simulink model "Torsional_System"  (R2021b)
settings: Solver=daessc  StartTime=0.0  StopTime=10.0  FixedStep=.001  RelTol=1e-3  AbsTol=1e-3  EnableMultiTasking=on
undefined symbols (not defined in the file or in its folder): X, Y, Z
libraries: sm_lib x119, nesl_utility x21, slpidlib x1
(part 1 of 6)
settings Model: Creator=HP Owner  LastModifiedBy=acontr14
settings SolverCC: AutoScaleAbsTol=off  AlgebraicLoopSolver=TrustRegion
settings DataIOCC: LimitDataPoints=on  MaxDataPoints=10000
settings OptimizationCC: LifeSpan=inf
settings DebuggingCC: AllowSymbolicDim=off  SFUnexpectedBacktrackingDiag=warning  SFNoUnconditionalDefaultTransitionDiag=warning  SFExecutionAtInitializationDiag=none  SFMachineParentedDataDiag=warning  ArithmeticOperatorsInVariantConditions=warning
settings SFSimCC: SimUseLocalCustomCode=off  CustomCodeUndefinedFunction=UseInterfaceOnly
settings RTWCC: RTWUseLocalCustomCode=off
settings CodeAppCC: StateflowObjectComments=on
settings GRTTargetCC: TargetLangStandard=C89/C90 (ANSI)
settings ConfigComp: CovMetricSettings=dw  CovSaveCumulativeToWorkspaceVar=on  CovSaveSingleToWorkspaceVar=on  CovExternalEMLEnable=off  CovSFcnEnable=off
settings SimscapeCC: SimscapeLogType=all  SimscapeLogSimulationStatistics=on  SimscapeLogDataHistory=10000
settings ExplorerConfigSet: InternalSimMechanicsExplorerSettings="<ExplorerConfiguration><canonicalview>default</canonicalview><AnimationSetting><BasePlaybackSpeed>1.0</BasePlaybackSpeed><PlaybackSpeedFactor>1.0</PlaybackSpeedFactor></AnimationSetting><TilePanel><TileInfo><Tiles Columns=\"1\" Count=\"1\" Rows=\"1\"><Column Weight=\"1\"/><Row Weight=\"1\"/><Tile Height=\"1\" Width=\"1\" X=\"0\" Y=\"0\"/></Tiles></TileInfo><SceneInfo><SceneViewer><BGColor><R>1</R><G>1</G><B>1</B></BGColor><Camera><DoPerspective>off</DoPerspective><Position><X>-0.306662978347955806</X><Y>-0.940894619780998753</Y><Z>0.41893568511161039</Z></Position><Center><X>-0.0242515964490015445</X><Y>-0.0315683410689719945</Y><Z>0.11337140346540675</Z></Center><Up><X>0.08382140599557307</X><Y>0.29392098737897232</Y><Z>0.9521472706861559</Z></Up><ViewLimDist>1</ViewLimDist><YLim>0.135911061057100324</YLim><XLim>0.110417778795510582</XLim></Camera></SceneViewer></SceneInfo></TilePanel><MechEditorPanel><Cameras/><GfxPanelCameraMap/><VideoCreator><PlaybackSpeedRatio>1.0</PlaybackSpeedRatio><FrameRate>30</FrameRate><VideoFormat>Motion JPEG AVI</VideoFormat><FrameSize>auto</FrameSize></VideoCreator></MechEditorPanel></ExplorerConfiguration>"

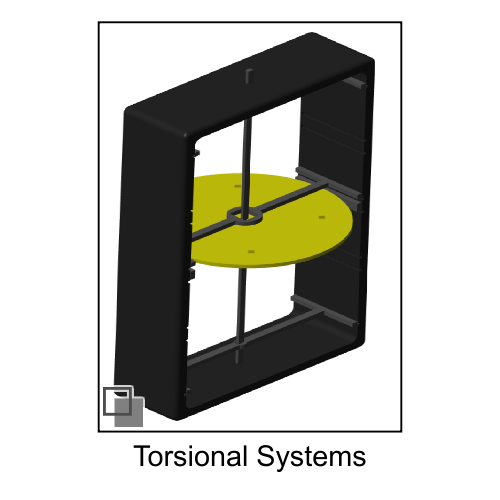
[thumbnail: Simulink's stored preview of the top-level diagram]
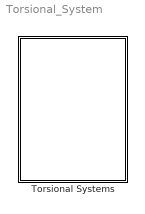
== system Torsional_System ==
  Torsional Systems : Subsystem  Variant=on  VariantControlMode=label  LabelModeActiveChoice=dof1PID

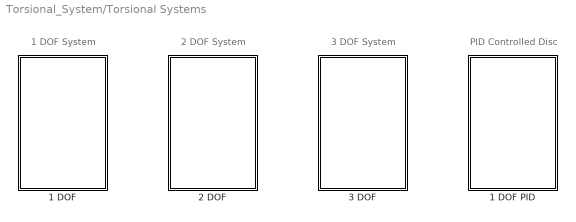
== system Torsional_System/Torsional Systems ==
  note: PID Controlled Disc
  note: 1 DOF System
  note: 2 DOF System
  note: 3 DOF System
  1 DOF : Subsystem  VariantControl=dof1  mask{materials=PLA, GG=3.5, b_den1=1.25, d_den=1.25, d=.000002, ll=106.800, load=off, lmass=5, dmass=15, pos1=50, zerodis=off, zero_forces=on, force_type=Harmonic, Force=2, Har_Force=2, freq=1}
      mask prompts: materials "Choose Material of Rod:"; GG "Shear Modulus (GPa):"; b_den1 "Density of Rod (g/cm^3):"; d_den "Density of Disc (g/cm^3):"; d "Rod Damping"; ll "Position of Disc (mm):"; load "Add load"; lmass "Load Mass (kg)"; dmass "Distance from Center (mm)"; pos1 "Initial Rotation of Disc (deg):"; zerodis "Zero Initial Displacement"; zero_forces "Zero Forces"; force_type "Force Response Type"; Force "Magnitude (N):"; Har_Force "Magnitude (N):"; freq "Frequency (rad/s):"
      mask init:
      | switch materials
      |     case 1
      |         G= 1; %GPa
      |         b_den= 1; %g/cm^3
      |     case 2
      |         G= 3.5;
      |         b_den= 1.24;
      |     case 3
      |         G= GG;
      |         b_den= b_den1;
      | end
      | switch force_type
      |     case 1
      |         Har_Force = 0;
      |         freq = 0;
      |     case 2
      |         Force = 0;
      | end
      | if zero_forces == 1
      |     Har_Force = 0;
      |     Force = 0;
      |     freq = 0;
      | end
      | if zerodis == 1
      |     pos1 = 0;
      | end
      | % l1=65e-3; l2=l1; l3=l1; l4=l1;
      | l=ll*10^-3;
      | l2=.2025-l;
      | G=G*10^9;
      | dd=2.25e-3;
      | k1=pi*G*dd^4/(32*l);
      | k2=(pi*G*dd^4/(32*l2));
      | % k3=(pi*G*dd^4/(32*l3));
      | kt1=k1+k2;
      | % kt2=k2+k3;
      | % kt3=2*k3;
      mask TypeOptions materials: Steel | PLA | Enter Material Properties
      mask Callback materials:
      | % Get the mask parameter values. This is a cell
      | %   array of character vectors.
      | maskStr = get_param(gcb,'materials');
      | 
      | % The pop-up menu is the first mask parameter.
      | %   Check the value selected in the pop-up
      | if strcmp(maskStr(1),'E'),
      | 
      |     % Set the visibility of both parameters on when
      |     %   User-defined is selected in the pop-up.
      | 
      |     set_param(gcb,'MaskVisibilities',{'on';'on';'on';'on';'on';'on';'on';'on';'on';'on';'on';'on';'on';'on';'on';'on'}),
      | 
      | else
      | 
      |     % Turn off the visibility of the Value field
      |     %   when User-defined is not selected.
      | 
      |     set_param(gcb,'MaskVisibilities',{'on';'off';'off';'on';'on';'on';'on';'on';'on';'on';'on';'on';'on';'on';'on';'on'}),
      | 
      |     % Set the character vector in the Values field equal to the
      |     % character vector selected in the Gain pop-up menu.
      | end
      mask Callback load:
      | load = get_param(gcb,'load');
      | if strcmp(load,'on')
      |     set_param('Torsional_System/Torsional Systems/1 DOF/Cylindrical Solid','Commented','off');
      |     set_param('Torsional_System/Torsional Systems/1 DOF/Rigid Transform2','Commented','off');
      | else
      |     set_param('Torsional_System/Torsional Systems/1 DOF/Cylindrical Solid','Commented','on');
      |     set_param('Torsional_System/Torsional Systems/1 DOF/Rigid Transform2','Commented','on');
      | end
      mask Callback zero_forces:
      | % Enable and disable parameters
      | 
      | % Get the value of the Enable Bias checkbox
      | % unchecked = 'off'
      | % checked = 'on'
      | enab = get_param(gcb,'zero_forces');
      | 
      | % Set the 'MaskEnables' property for each parameters
      | if strcmp(enab,'on')
      |     set_param(gcb,'MaskEnables',{'on','on','on','on','on','on','on','on','on','on','on','on','off','off','off','off'});
      | else
      |     set_param(gcb,'MaskEnables',{'on','on','on','on','on','on','on','on','on','on','on','on','on','on','on','on'});
      | end
      | 
      | % Note that the value of the bias is not handled here.
      | % See the Initialization tab
      mask TypeOptions force_type: Step | Harmonic
      mask DialogControl Control4 Prompt: Update Model
      mask DialogControl Control4 Callback: set_param(bdroot,'SimulationCommand','update')
      mask DialogControl Control3 Prompt: Run Simulation
      mask DialogControl Control3 Callback: set_param(bdroot,'SimulationCommand','start')
      mask DialogControl Control5 Prompt: Stop Simulation
      mask DialogControl Control5 Callback: set_param(bdroot,'SimulationCommand','stop')
      mask DialogControl Control2 Prompt: Open Position Plot
      mask DialogControl Control2 Callback: open(Simulink.BlockPath({'Torsional_System/Torsional Systems/1 DOF/Scope1'}))
      mask DialogControl Control7 Prompt: Open Frequency Plot
      mask DialogControl Control7 Callback:
      | disc1=evalin('base','out.disc1_pos');
      | time=evalin('base','out.tout');
      | 
      | Ts = time(2)-time(1);
      | fs = 1/Ts;
      | N = length(disc1);
      | 
      | Y1 = abs(fft(disc1)/N); % fft of cart1 data
      | Y1d = Y1(1:N/2+1); %single side spectrum
      | Y1d(2:end-1) = 2*Y1d(2:end-1); %amplitude adjustment
      | 
      | f = fs*(0:(N/2))/N; %create frequency vector
      | 
      | figure;
      | plot(f,Y1d); xlim([0 10]);
      mask DialogControl Container8 Prompt: Parameters
      mask DialogControl Container14 Prompt: Loading
      mask DialogControl Container13 Prompt: Free Response
      mask DialogControl Container17 Prompt: Force Response
      mask DialogControl Container18 Prompt: Step Response
      mask DialogControl Container19 Prompt: Harmonic Response
      mask Display: image('$imagefile'); % Use "Edit Image" on toolstrip to change.
  1 DOF PID : Subsystem  VariantControl=dof1PID  mask{materials=PLA, GG=3.5, b_den1=1.25, d_den=1.25, d=.000002, ll=106.800, load=off, lmass=5, dmass=37.0, pos1=50, zerodis=on, zero_forces=off, force_type=Pulse, Force=5, Har_Force=2, freq=1, Pulse_Force=2, Pulse_Period=3, Pulse_Width=5, PID_source=Square, sin_amp=30, sin_freq=1, squ_amp=50, squ_freq=.2, step_mag=30}
      mask prompts: materials "Choose Material of Rod:"; GG "Shear Modulus (GPa):"; b_den1 "Density of Rod (g/cm^3):"; d_den "Density of Disc (g/cm^3):"; d "Rod Damping"; ll "Position of Disc (mm):"; load "Add Load"; lmass "Load Mass (kg)"; dmass "Distance from Center (mm)"; pos1 "Initial Rotation of Disc (deg):"; zerodis "Zero Initial Displacement"; zero_forces "Zero Forces"; force_type "Force Response Type"; Force "Magnitude (N):"; Har_Force "Magnitude (N):"; freq "Frequency (rad/s):"; Pulse_Force "Magnitude (N):"; Pulse_Period "Period (sec):"; Pulse_Width "Pulse Width (% of period):"; PID_source "Angle Signal"; sin_amp "Amplitude (deg):"; sin_freq "Frequency (rad/sec):"; squ_amp "Amplitude (deg):"; squ_freq "Frequency (Hz):"; step_mag "Magnitude (deg):"
      mask init:
      | switch materials
      |     case 1
      |         G= 1; %GPa
      |         b_den= 1; %g/cm^3
      |     case 2
      |         G= 3.5;
      |         b_den= 1.24;
      |     case 3
      |         G= GG;
      |         b_den= b_den1;
      | end
      | switch force_type
      |     case 1
      |         Har_Force = 0;
      |         freq = 0;
      |         Pulse_Force = 0;
      |     case 2
      |         Force = 0;
      |         Pulse_Force = 0;
      |     case 3
      |         Har_Force = 0;
      |         freq = 0;
      |         Force = 0;
      | end
      | if zero_forces == 1
      |     Har_Force = 0;
      |     Force = 0;
      |     freq = 0;
      | end
      | if zerodis == 1
      |     pos1 = 0;
      | end
      | switch PID_source
      |     case 1
      |         set_param('Torsional_System/Torsional Systems/1 DOF PID/Sine Wave2','Commented','off');
      |         set_param('Torsional_System/Torsional Systems/1 DOF PID/Signal Generator','Commented','on');
      |         set_param('Torsional_System/Torsional Systems/1 DOF PID/Step2','Commented','on');
      |     case 2
      |         set_param('Torsional_System/Torsional Systems/1 DOF PID/Sine Wave2','Commented','on');
      |         set_param('Torsional_System/Torsional Systems/1 DOF PID/Signal Generator','Commented','off');
      |         set_param('Torsional_System/Torsional Systems/1 DOF PID/Step2','Commented','on');
      |     case 3
      |         set_param('Torsional_System/Torsional Systems/1 DOF PID/Sine Wave2','Commented','on');
      |         set_param('Torsional_System/Torsional Systems/1 DOF PID/Signal Generator','Commented','on');
      |         set_param('Torsional_System/Torsional Systems/1 DOF PID/Step2','Commented','off');
      | end
      | % l1=65e-3; l2=l1; l3=l1; l4=l1;
      | l=ll*10^-3;
      | l2=.2025-l;
      | G=G*10^9;
      | dd=2.25e-3;
      | k1=pi*G*dd^4/(32*l);
      | k2=(pi*G*dd^4/(32*l2));
      | % k3=(pi*G*dd^4/(32*l3));
      | kt1=k1+k2;
      | % kt2=k2+k3;
      | % kt3=2*k3;
      mask TypeOptions materials: Steel | PLA | Enter Material Properties
      mask Callback materials:
      | % Get the mask parameter values. This is a cell
      | %   array of character vectors.
      | maskStr = get_param(gcb,'materials');
      | 
      | % The pop-up menu is the first mask parameter.
      | %   Check the value selected in the pop-up
      | if strcmp(maskStr(1),'E'),
      | 
      |     % Set the visibility of both parameters on when
      |     %   User-defined is selected in the pop-up.
      | 
      |     set_param(gcb,'MaskVisibilities',{'on';'on';'on';'on';'on';'on';'on';'on';'on';'on';'on';'on';'on';'on';'on';'on';'on';'on';'on';'on';'on';'on';'on';'on';'on'}),
      | 
      | else
      | 
      |     % Turn off the visibility of the Value field
      |     %   when User-defined is not selected.
      | 
      |     set_param(gcb,'MaskVisibilities',{'on';'off';'off';'on';'on';'on';'on';'on';'on';'on';'on';'on';'on';'on';'on';'on';'on';'on';'on';'on';'on';'on';'on';'on';'on'}),
      | 
      |     % Set the character vector in the Values field equal to the
      |     % character vector selected in the Gain pop-up menu.
      | end
      mask Callback load:
      | load = get_param(gcb,'load');
      | if strcmp(load,'on')
      |     set_param('Torsional_System/Torsional Systems/1 DOF PID/Cylindrical Solid','Commented','off');
      |     set_param('Torsional_System/Torsional Systems/1 DOF PID/Rigid Transform9','Commented','off');
      |     set_param('Torsional_System/Torsional Systems/1 DOF PID/Cylindrical Solid1','Commented','off');
      |     set_param('Torsional_System/Torsional Systems/1 DOF PID/Rigid Transform7','Commented','off');
      | else
      |     set_param('Torsional_System/Torsional Systems/1 DOF PID/Cylindrical Solid','Commented','on');
      |     set_param('Torsional_System/Torsional Systems/1 DOF PID/Rigid Transform9','Commented','on');
      |     set_param('Torsional_System/Torsional Systems/1 DOF PID/Cylindrical Solid1','Commented','on');
      |     set_param('Torsional_System/Torsional Systems/1 DOF PID/Rigid Transform7','Commented','on');
      | end
      mask Callback zero_forces:
      | % Enable and disable parameters
      | 
      | % Get the value of the Enable Bias checkbox
      | % unchecked = 'off'
      | % checked = 'on'
      | enab = get_param(gcb,'zero_forces');
      | 
      | % Set the 'MaskEnables' property for each parameters
      | if strcmp(enab,'on')
      |     set_param(gcb,'MaskEnables',{'on','on','on','on','on','on','on','on','on','on','on','on','off','off','off','off','off','off','off','on','on','on','on','on','on'});
      | else
      |     set_param(gcb,'MaskEnables',{'on','on','on','on','on','on','on','on','on','on','on','on','on','on','on','on','on','on','on','on','on','on','on','on','on'});
      | end
      | 
      | % Note that the value of the bias is not handled here.
      | % See the Initialization tab
      mask TypeOptions force_type: Step | Harmonic | Pulse
      mask TypeOptions PID_source: Harmonic | Square | Constant
      mask DialogControl Control4 Prompt: Update Model
      mask DialogControl Control4 Callback: set_param(bdroot,'SimulationCommand','update')
      mask DialogControl Control3 Prompt: Run Simulation
      mask DialogControl Control3 Callback: set_param(bdroot,'SimulationCommand','start')
      mask DialogControl Control5 Prompt: Stop Simulation
      mask DialogControl Control5 Callback: set_param(bdroot,'SimulationCommand','stop')
      mask DialogControl Control2 Prompt: Open Position Plot
      mask DialogControl Control2 Callback: open(Simulink.BlockPath({'Torsional_System/Torsional Systems/1 DOF PID/Scope1'}))
      mask DialogControl Control7 Prompt: Open PID Controller
      mask DialogControl Control7 Callback: open(Simulink.BlockPath({'Torsional_System/Torsional Systems/1 DOF PID/PID Controller'}))
      mask DialogControl Container8 Prompt: Parameters
      mask DialogControl Container14 Prompt: Loading
      mask DialogControl Container13 Prompt: Free Response
      mask DialogControl Container17 Prompt: Force Response
      mask DialogControl Container18 Prompt: Step Response
      mask DialogControl Container19 Prompt: Harmonic Response
      mask DialogControl Container23 Prompt: Pulse
      mask DialogControl Container16 Prompt: PID Desired Angle
      mask DialogControl Container20 Prompt: Harmonic
      mask DialogControl Container21 Prompt: Square
      mask DialogControl Container22 Prompt: Constant
      mask Display: image('$imagefile'); % Use "Edit Image" on toolstrip to change.
  2 DOF : Subsystem  VariantControl=dof2  mask{materials=PLA, GG=3.5, b_den1=1.25, d_den=1.25, d=.000002, ll1=45.600, ll2=163.0, load=off, lmass=5, dmass=15, pos1=15, pos2=30, zerodis=off, zero_forces=on, force_type=Step, Force_m1=0, Force_m2=0, Har_Force_m1=0, freq_m1=0, Har_Force_m2=0, freq_m2=0}
      mask prompts: materials "Choose Material of Rod:"; GG "Shear Modulus (GPa):"; b_den1 "Density of Rod (g/cm^3):"; d_den "Density of Discs (g/cm^3):"; d "Rod Damping"; ll1 "Position of Disc 1 (mm):"; ll2 "Position of Disc 2 (mm):"; load "Add load"; lmass "Load Mass (kg)"; dmass "Distance from Center (mm)"; pos1 "Initial Rotation of Disc 1 (deg):"; pos2 "Initial Rotation of Disc 2 (deg):"; zerodis "Zero Initial Displacement"; zero_forces "Zero Forces"; force_type "Force Response Type"; Force_m1 "Magnitude  on Disc 1 (N):"; Force_m2 "Magnitude  on Disc 2 (N):"; Har_Force_m1 "Magnitude on Disc 1 (N):"; freq_m1 "Frequency on Disc 1 (rad/s):"; Har_Force_m2 "Magnitude on Disc 2 (N):"; freq_m2 "Frequency on Disc 2 (rad/s):"
      mask init:
      | switch materials
      |     case 1
      |         G= 1; %GPa
      |         b_den= 1; %g/cm^3
      |     case 2
      |         G= 3.5;
      |         b_den= 1.24;
      |     case 3
      |         G= GG;
      |         b_den= b_den1;
      | end
      | switch force_type
      |     case 1
      |         Har_Force_m1 = 0;
      |         freq_m1 = 0;
      |         Har_Force_m2 = 0;
      |         freq_m2 = 0;
      |     case 2
      |         Force_m1 = 0;
      |         Force_m2 = 0;
      | end
      | if zero_forces == 1
      |     Har_Force_m1 = 0;
      |     freq_m1 = 0;
      |     Har_Force_m2 = 0;
      |     freq_m2 = 0;
      |     Force_m1 = 0;
      |     Force_m2 = 0;
      | end
      | if zerodis == 1
      |     pos1 = 0;
      |     pos2 = 0;
      | end
      | l1=ll1*10^-3;
      | l2=ll2*10^-3;
      | l2=l2-l1;
      | l3=202.5-(ll2*10^-3);
      | G=G*10^9;
      | dd=2.25e-3;
      | k1=pi*G*dd^4/(32*l1);
      | k2=(pi*G*dd^4/(32*l2));
      | k3=(pi*G*dd^4/(32*l3));
      | kt1=k1+k2;
      | kt2=k2+k3;
      mask TypeOptions materials: Steel | PLA | Enter Material Properties
      mask Callback materials:
      | % Get the mask parameter values. This is a cell
      | %   array of character vectors.
      | maskStr = get_param(gcb,'materials');
      | 
      | % The pop-up menu is the first mask parameter.
      | %   Check the value selected in the pop-up
      | if strcmp(maskStr(1),'E'),
      | 
      |     % Set the visibility of both parameters on when
      |     %   User-defined is selected in the pop-up.
      | 
      |     set_param(gcb,'MaskVisibilities',{'on';'on';'on';'on';'on';'on';'on';'on';'on';'on';'on';'on';'on';'on';'on';'on';'on';'on';'on';'on';'on'}),
      | 
      | else
      | 
      |     % Turn off the visibility of the Value field
      |     %   when User-defined is not selected.
      | 
      |     set_param(gcb,'MaskVisibilities',{'on';'off';'off';'on';'on';'on';'on';'on';'on';'on';'on';'on';'on';'on';'on';'on';'on';'on';'on';'on';'on'}),
      | 
      |     % Set the character vector in the Values field equal to the
      |     % character vector selected in the Gain pop-up menu.
      | end
      mask Callback load:
      | load = get_param(gcb,'load');
      | if strcmp(load,'on')
      |     set_param('Torsional_System/Torsional Systems/2 DOF/Cylindrical Solid','Commented','off');
      |     set_param('Torsional_System/Torsional Systems/2 DOF/Rigid Transform6','Commented','off');
      |     set_param('Torsional_System/Torsional Systems/2 DOF/Cylindrical Solid1','Commented','off');
      |     set_param('Torsional_System/Torsional Systems/2 DOF/Rigid Transform7','Commented','off');
      | else
      |     set_param('Torsional_System/Torsional Systems/2 DOF/Cylindrical Solid','Commented','on');
      |     set_param('Torsional_System/Torsional Systems/2 DOF/Rigid Transform6','Commented','on');
      |     set_param('Torsional_System/Torsional Systems/2 DOF/Cylindrical Solid1','Commented','on');
      |     set_param('Torsional_System/Torsional Systems/2 DOF/Rigid Transform7','Commented','on');
      | end
      mask Callback zero_forces:
      | % Enable and disable parameters
      | 
      | % Get the value of the Enable Bias checkbox
      | % unchecked = 'off'
      | % checked = 'on'
      | enab = get_param(gcb,'zero_forces');
      | 
      | % Set the 'MaskEnables' property for each parameters
      | if strcmp(enab,'on')
      |     set_param(gcb,'MaskEnables',{'on','on','on','on','on','on','on','on','on','on','on','on','on','on','off','off','off','off','off','off','off'});
      | else
      |     set_param(gcb,'MaskEnables',{'on','on','on','on','on','on','on','on','on','on','on','on','on','on','on','on','on','on','on','on','on'});
      | end
      | 
      | % Note that the value of the bias is not handled here.
      | % See the Initialization tab
      mask TypeOptions force_type: Step | Harmonic
      mask DialogControl Control4 Prompt: Update Model
      mask DialogControl Control4 Callback: set_param(bdroot,'SimulationCommand','update')
      mask DialogControl Control3 Prompt: Run Simulation
      mask DialogControl Control3 Callback: set_param(bdroot,'SimulationCommand','start')
      mask DialogControl Control5 Prompt: Stop Simulation
      mask DialogControl Control5 Callback: set_param(bdroot,'SimulationCommand','stop')
      mask DialogControl Control2 Prompt: Open Position Plot
      mask DialogControl Control2 Callback: open(Simulink.BlockPath({'Torsional_System/Torsional Systems/2 DOF/Scope1'}))
      mask DialogControl Control7 Prompt: Open Frequency Plot
      mask DialogControl Control7 Callback:
      | disc1=evalin('base','out.disc1_pos');
      | disc2=evalin('base','out.disc2_pos');
      | time=evalin('base','out.tout');
      | 
      | Ts = time(2)-time(1);
      | fs = 1/Ts;
      | N = length(disc1);
      | 
      | Y1 = abs(fft(disc1)/N); % fft of cart1 data
      | Y1d = Y1(1:N/2+1); %single side spectrum
      | Y1d(2:end-1) = 2*Y1d(2:end-1); %amplitude adjustment
      | 
      | Y2 = abs(fft(disc2)/N);
      | Y2d = Y2(1:N/2+1);
      | Y2d(2:end-1) = 2*Y2d(2:end-1);
      | 
      | 
      | f = fs*(0:(N/2))/N; %create frequency vector
      | 
      | figure;
      | plot(f,Y1d); xlim([0 10]);
      | hold on;
      | plot(f,Y2d,'r')
      | hold off;
      mask DialogControl Container10 Prompt: Parameters
      mask DialogControl Container17 Prompt: Loading
      mask DialogControl Container11 Prompt: Free Response
      mask DialogControl Container12 Prompt: Forced Response
      mask DialogControl Container15 Prompt: Step Response
      mask DialogControl Container16 Prompt: Harmonic Response
      mask Display: image('$imagefile'); % Use "Edit Image" on toolstrip to change.
  3 DOF : Subsystem  VariantControl=dof3  mask{materials=Steel, GG=3.5, b_den1=1.25, d_den=1.25, d=.000002, ll1=45.150, ll2=106.500, ll3=163.850, load=off, lmass=5, dmass=15, pos1=30, pos2=30, pos3=30, zerodis=off, zero_forces=on, force_type=Step, Force_m1=0, Force_m2=0, Force_m3=0, Har_Force_m1=0, freq_m1=0, Har_Force_m2=0, freq_m2=0, Har_Force_m3=0, freq_m3=0}
      mask prompts: materials "Choose Material of Rod:"; GG "Shear Modulus (GPa):"; b_den1 "Density of Rod (g/cm^3):"; d_den "Density of Discs (g/cm^3):"; d "Rod Damping"; ll1 "Position of Disc 1 (mm):"; ll2 "Position of Disc 2 (mm):"; ll3 "Position of Disc 3 (mm):"; load "Add Load"; lmass "Load Mass (kg)"; dmass "Distance from Center (mm)"; pos1 "Initial Rotation of Disc 1 (deg):"; pos2 "Initial Rotation of Disc 2 (deg):"; pos3 "Initial Rotation of Disc (deg):"; zerodis "Zero Initial Displacement"; zero_forces "Zero Forces"; force_type "Force Type"; Force_m1 "Magnitude  on Disc 1 (N):"; Force_m2 "Magnitude  on Disc 2 (N):"; Force_m3 "Magnitude  on Disc 3 (N):"; Har_Force_m1 "Magnitude on Disc 1 (N):"; freq_m1 "Frequency on Disc 1 (rad/s):"; Har_Force_m2 "Magnitude on Disc 2 (N):"; freq_m2 "Frequency on Disc 2 (rad/s):"; Har_Force_m3 "Magnitude on Disc 3 (N):"; freq_m3 "Frequency on Disc 3 (rad/s):"
      mask init:
      | switch materials
      |     case 1
      |         G= 1; %GPa
      |         b_den= 1; %g/cm^3
      |     case 2
      |         G= 3.5;
      |         b_den= 1.24;
      |     case 3
      |         G= GG;
      |         b_den= b_den1;
      | end
      | switch force_type
      |     case 1
      |         Har_Force_m1 = 0;
      |         freq_m1 = 0;
      |         Har_Force_m2 = 0;
      |         freq_m2 = 0;
      |         Har_Force_m3 = 0;
      |         freq_m3 = 0;
      |     case 2
      |         Force_m1 = 0;
      |         Force_m2 = 0;
      |         Force_m3 = 0;
      | end
      | if zero_forces == 1
      |     Har_Force_m1 = 0;
      |     freq_m1 = 0;
      |     Har_Force_m2 = 0;
      |     freq_m2 = 0;
      |     Har_Force_m3 = 0;
      |     freq_m3 = 0;
      |     Force_m1 = 0;
      |     Force_m2 = 0;
      |     Force_m3 = 0;
      | end
      | if zerodis == 1
      |     pos1 = 0;
      |     pos2 = 0;
      |     pos3 = 0;
      | end
      | l1=ll1*10^-3;
      | l2=ll2*10^-3;
      | l3=ll3*10^-3;
      | l2=l2-l1;
      | l3=l3-(ll2*10^-3);
      | l4=202.5-(ll3*10^-3);
      | G=G*10^9;
      | dd=2.25e-3;
      | k1=pi*G*dd^4/(32*l1);
      | k2=(pi*G*dd^4/(32*l2));
      | k3=(pi*G*dd^4/(32*l3));
      | k4=(pi*G*dd^4/(32*l4));
      | kt1=k1+k2;
      | kt2=k2+k3;
      | kt3=k3+k4;
      mask TypeOptions materials: Steel | PLA | Enter Material Properties
      mask Callback materials:
      | % Get the mask parameter values. This is a cell
      | %   array of character vectors.
      | maskStr = get_param(gcb,'materials');
      | 
      | % The pop-up menu is the first mask parameter.
      | %   Check the value selected in the pop-up
      | if strcmp(maskStr(1),'E'),
      | 
      |     % Set the visibility of both parameters on when
      |     %   User-defined is selected in the pop-up.
      | 
      |     set_param(gcb,'MaskVisibilities',{'on';'on';'on';'on';'on';'on';'on';'on';'on';'on';'on';'on';'on';'on';'on';'on';'on';'on';'on';'on';'on';'on';'on';'on';'on';'on'}),
      | 
      | else
      | 
      |     % Turn off the visibility of the Value field
      |     %   when User-defined is not selected.
      | 
      |     set_param(gcb,'MaskVisibilities',{'on';'off';'off';'on';'on';'on';'on';'on';'on';'on';'on';'on';'on';'on';'on';'on';'on';'on';'on';'on';'on';'on';'on';'on';'on';'on'}),
      | 
      |     % Set the character vector in the Values field equal to the
      |     % character vector selected in the Gain pop-up menu.
      | end
      mask Callback load:
      | load = get_param(gcb,'load');
      | if strcmp(load,'on')
      |     set_param('Torsional_System/Torsional Systems/3 DOF/Cylindrical Solid','Commented','off');
      |     set_param('Torsional_System/Torsional Systems/3 DOF/Rigid Transform9','Commented','off');
      |     set_param('Torsional_System/Torsional Systems/3 DOF/Cylindrical Solid1','Commented','off');
      |     set_param('Torsional_System/Torsional Systems/3 DOF/Rigid Transform10','Commented','off');
      |     set_param('Torsional_System/Torsional Systems/3 DOF/Cylindrical Solid2','Commented','off');
      |     set_param('Torsional_System/Torsional Systems/3 DOF/Rigid Transform11','Commented','off');
      | else
      |     set_param('Torsional_System/Torsional Systems/3 DOF/Cylindrical Solid','Commented','on');
      |     set_param('Torsional_System/Torsional Systems/3 DOF/Rigid Transform9','Commented','on');
      |     set_param('Torsional_System/Torsional Systems/3 DOF/Cylindrical Solid1','Commented','on');
      |     set_param('Torsional_System/Torsional Systems/3 DOF/Rigid Transform10','Commented','on');
      |     set_param('Torsional_System/Torsional Systems/3 DOF/Cylindrical Solid2','Commented','on');
      |     set_param('Torsional_System/Torsional Systems/3 DOF/Rigid Transform11','Commented','on');
      | end
      mask Callback zero_forces:
      | % Enable and disable parameters
      | 
      | % Get the value of the Enable Bias checkbox
      | % unchecked = 'off'
      | % checked = 'on'
      | enab = get_param(gcb,'zero_forces');
      | 
      | % Set the 'MaskEnables' property for each parameters
      | if strcmp(enab,'on')
      |     set_param(gcb,'MaskEnables',{'on','on','on','on','on','on','on','on','on','on','on','on','on','on','on','on','off','off','off','off','off','off','off','off','off','off'});
      | else
      |     set_param(gcb,'MaskEnables',{'on','on','on','on','on','on','on','on','on','on','on','on','on','on','on','on','on','on','on','on','on','on','on','on','on','on'});
      | end
      | 
      | % Note that the value of the bias is not handled here.
      | % See the Initialization tab
      mask TypeOptions force_type: Step | Harmonic
      mask DialogControl Control4 Prompt: Update Model
      mask DialogControl Control4 Callback: set_param(bdroot,'SimulationCommand','update')
      mask DialogControl Control3 Prompt: Run Simulation
      mask DialogControl Control3 Callback: set_param(bdroot,'SimulationCommand','start')
      mask DialogControl Control5 Prompt: Stop Simulation
      mask DialogControl Control5 Callback: set_param(bdroot,'SimulationCommand','stop')
      mask DialogControl Control2 Prompt: Open Position Plot
      mask DialogControl Control2 Callback: open(Simulink.BlockPath({'Torsional_System/Torsional Systems/3 DOF/Scope1'}))
      mask DialogControl Control7 Callback:
      | disc1=evalin('base','out.disc1_pos');
      | disc2=evalin('base','out.disc2_pos');
      | disc3=evalin('base','out.disc3_pos');
      | time=evalin('base','out.tout');
      | 
      | Ts = time(2)-time(1);
      | fs = 1/Ts;
      | N = length(disc1);
      | 
      | Y1 = abs(fft(disc1)/N); % fft of cart1 data
      | Y1d = Y1(1:N/2+1); %single side spectrum
      | Y1d(2:end-1) = 2*Y1d(2:end-1); %amplitude adjustment
      | 
      | Y2 = abs(fft(disc2)/N);
      | Y2d = Y2(1:N/2+1);
      | Y2d(2:end-1) = 2*Y2d(2:end-1);
      | 
      | Y3 = abs(fft(disc3)/N);
      | Y3d = Y3(1:N/2+1);
      | Y3d(2:end-1) = 2*Y3d(2:end-1);
      | 
      | 
      | f = fs*(0:(N/2))/N; %create frequency vector
      | 
      | figure;
      | plot(f,Y1d); xlim([0 10]);
      | hold on;
      | plot(f,Y2d,'r')
      | plot(f,Y3d,'g')
      | hold off;
      mask DialogControl Container8 Prompt: Parameters
      mask DialogControl Container14 Prompt: Loading
      mask DialogControl Container9 Prompt: Free Response
      mask DialogControl Container10 Prompt: Forced Response
      mask DialogControl Container11 Prompt: Step
      mask DialogControl Container12 Prompt: Harmonic
      mask Display: image('$imagefile'); % Use "Edit Image" on toolstrip to change.

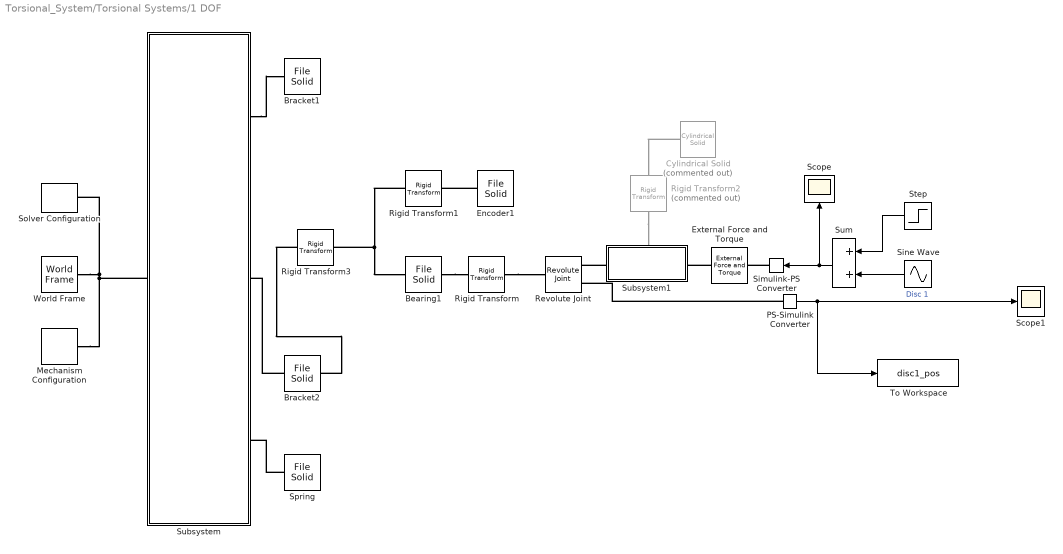
== system Torsional_System/Torsional Systems/1 DOF ==
  Bearing1 : sm_lib/Body Elements/File Solid  ExtGeomFileName=TS-Bearing 2.0_Default_sldprt.STEP  UnitType=FromFile  ExtGeomFileUnits=m  StepReaderType=HEX  ExportConvexHullGeometry=off  InertiaType=CalculateFromGeometry  Mass=1  MassUnits=kg  CenterOfMass=[0 0 0]  CenterOfMassUnits=m  MomentsOfInertia=[1 1 1]  MomentsOfInertiaUnits=kg*m^2  ProductsOfInertia=[0 0 0]  ProductsOfInertiaUnits=kg*m^2  BasedOnType=Density  Density=1000  DensityUnits=kg/m^3  DoExposeReferenceFrame=off  SerializedFrames=<Frames><Frame><Id>Frame1</Id><Value><Name>F1</Name><Origin><Source>GeometricFeature</Source><FeatureName>planar surface 2</FeatureName></Origin><PrimaryAxis><DefinedDirection>+Z</DefinedDirection><Source>ReferenceFrame</Source><SourceDirection>+Z</SourceDirection><FeatureName></FeatureName></PrimaryAxis><SecondaryAxis><DefinedDirection>+X</DefinedDirection><Source>ReferenceFrame</Source><SourceDirection>+X</SourceDirection><FeatureName></FeatureName></SecondaryAxis></Value></Frame><Frame><Id>Frame3</Id><Value><Name>bearing_bottom</Name><Origin><Source>GeometricFeature</Source><FeatureName>circular curve 14</FeatureName></Origin><PrimaryAxis><DefinedDirection>+Z</DefinedDirection><Source>ReferenceFrame</Source><SourceDirection>+Z</SourceDirection><FeatureName></FeatureName></PrimaryAxis><SecondaryAxis><DefinedDirection>+X</DefinedDirection><Source>ReferenceFrame</Source><SourceDirection>+X</SourceDirection><FeatureName></FeatureName></SecondaryAxis></Value></Frame></Frames>  GraphicType=FromGeometry  MarkerShape=Sphere  MarkerSize=10  GraphicVisPropType=SimpleVisualProperties  GraphicDiffuseColor=[0.4 0.4 0.4]  GraphicSpecularColor=[0.5 0.5 0.5 1.0]  GraphicAmbientColor=[0.15 0.15 0.15 1.0]  GraphicEmissiveColor=[0.0 0.0 0.0 1.0]  GraphicShininess=75  GraphicOpacity=1
  Bracket1 : sm_lib/Body Elements/File Solid  ExtGeomFileName=TS-Bracket 2.0_Default_sldprt.STEP  UnitType=FromFile  ExtGeomFileUnits=m  StepReaderType=HEX  ExportConvexHullGeometry=off  InertiaType=CalculateFromGeometry  Mass=1  MassUnits=kg  CenterOfMass=[0 0 0]  CenterOfMassUnits=m  MomentsOfInertia=[1 1 1]  MomentsOfInertiaUnits=kg*m^2  ProductsOfInertia=[0 0 0]  ProductsOfInertiaUnits=kg*m^2  BasedOnType=Density  Density=1000  DensityUnits=kg/m^3  DoExposeReferenceFrame=off  SerializedFrames=<Frames><Frame><Id>Frame1</Id><Value><Name>F1</Name><Origin><Source>GeometricFeature</Source><FeatureName>planar surface 4</FeatureName></Origin><PrimaryAxis><DefinedDirection>+Z</DefinedDirection><Source>ReferenceFrame</Source><SourceDirection>+Z</SourceDirection><FeatureName></FeatureName></PrimaryAxis><SecondaryAxis><DefinedDirection>+X</DefinedDirection><Source>ReferenceFrame</Source><SourceDirection>+X</SourceDirection><FeatureName></FeatureName></SecondaryAxis></Value></Frame><Frame><Id>Frame2</Id><Value><Name>F2</Name><Origin><Source>GeometricFeature</Source><FeatureName>planar surface 11</FeatureName></Origin><PrimaryAxis><DefinedDirection>+Z</DefinedDirection><Source>ReferenceFrame</Source><SourceDirection>+Z</SourceDirection><FeatureName></FeatureName></PrimaryAxis><SecondaryAxis><DefinedDirection>+X</DefinedDirection><Source>ReferenceFrame</Source><SourceDirection>+X</SourceDirection><FeatureName></FeatureName></SecondaryAxis></Value></Frame></Frames>  GraphicType=FromGeometry  MarkerShape=Sphere  MarkerSize=10  GraphicVisPropType=SimpleVisualProperties  GraphicDiffuseColor=[0.4 0.4 0.4]  GraphicSpecularColor=[0.5 0.5 0.5 1.0]  GraphicAmbientColor=[0.15 0.15 0.15 1.0]  GraphicEmissiveColor=[0.0 0.0 0.0 1.0]  GraphicShininess=75  GraphicOpacity=1
  Bracket2 : sm_lib/Body Elements/File Solid  ExtGeomFileName=TS-Bracket 2.0_Default_sldprt.STEP  UnitType=FromFile  ExtGeomFileUnits=m  StepReaderType=HEX  ExportConvexHullGeometry=off  InertiaType=CalculateFromGeometry  Mass=1  MassUnits=kg  CenterOfMass=[0 0 0]  CenterOfMassUnits=m  MomentsOfInertia=[1 1 1]  MomentsOfInertiaUnits=kg*m^2  ProductsOfInertia=[0 0 0]  ProductsOfInertiaUnits=kg*m^2  BasedOnType=Density  Density=1000  DensityUnits=kg/m^3  DoExposeReferenceFrame=off  SerializedFrames=<Frames><Frame><Id>Frame1</Id><Value><Name>F1</Name><Origin><Source>GeometricFeature</Source><FeatureName>planar surface 4</FeatureName></Origin><PrimaryAxis><DefinedDirection>+Z</DefinedDirection><Source>ReferenceFrame</Source><SourceDirection>+Z</SourceDirection><FeatureName></FeatureName></PrimaryAxis><SecondaryAxis><DefinedDirection>+X</DefinedDirection><Source>ReferenceFrame</Source><SourceDirection>+X</SourceDirection><FeatureName></FeatureName></SecondaryAxis></Value></Frame><Frame><Id>Frame2</Id><Value><Name>F2</Name><Origin><Source>GeometricFeature</Source><FeatureName>planar surface 4</FeatureName></Origin><PrimaryAxis><DefinedDirection>+Z</DefinedDirection><Source>ReferenceFrame</Source><SourceDirection>+Z</SourceDirection><FeatureName></FeatureName></PrimaryAxis><SecondaryAxis><DefinedDirection>+X</DefinedDirection><Source>ReferenceFrame</Source><SourceDirection>+X</SourceDirection><FeatureName></FeatureName></SecondaryAxis></Value></Frame></Frames>  GraphicType=FromGeometry  MarkerShape=Sphere  MarkerSize=10  GraphicVisPropType=SimpleVisualProperties  GraphicDiffuseColor=[0.4 0.4 0.4]  GraphicSpecularColor=[0.5 0.5 0.5 1.0]  GraphicAmbientColor=[0.15 0.15 0.15 1.0]  GraphicEmissiveColor=[0.0 0.0 0.0 1.0]  GraphicShininess=75  GraphicOpacity=1
  Cylindrical Solid : sm_lib/Body Elements/Cylindrical Solid  Commented=on  GraphicAmbientColor=[0.15 0.15 0.15 1.0]  BasedOnType=Mass  CenterOfMass=[0 0 0]  CenterOfMassUnits=m  GraphicDiffuseColor=[0.18039216 0.18039216 0.18039216]  CylinderLength=.5  CylinderLengthUnits=cm  CylinderRadius=.5  CylinderRadiusUnits=cm  Density=1000  DensityUnits=kg/m^3  DoExposeReferenceFrame=off  GraphicEmissiveColor=[0.0 0.0 0.0 1.0]  ExportEntireGeometry=off  SerializedFrames=<Frames><Frame><Id>Frame1</Id><Value><Name>F1</Name><Origin><Source>GeometricFeature</Source><FeatureName>bottom surface</FeatureName></Origin><PrimaryAxis><DefinedDirection>+Z</DefinedDirection><Source>ReferenceFrame</Source><SourceDirection>+Z</SourceDirection><FeatureName></FeatureName></PrimaryAxis><SecondaryAxis><DefinedDirection>+X</DefinedDirection><Source>ReferenceFrame</Source><SourceDirection>+X</SourceDirection><FeatureName></FeatureName></SecondaryAxis></Value></Frame></Frames>  MarkerShape=Sphere  MarkerSize=10  GraphicType=FromGeometry  InertiaType=CalculateFromGeometry  Mass=lmass  MassUnits=kg  MomentsOfInertia=[1 1 1]  MomentsOfInertiaUnits=kg*m^2  GraphicOpacity=1.0  ProductsOfInertia=[0 0 0]  ProductsOfInertiaUnits=kg*m^2  GraphicShininess=75  GraphicSpecularColor=[0.5 0.5 0.5 1.0]  GraphicVisPropType=SimpleVisualProperties
  Encoder1 : sm_lib/Body Elements/File Solid  ExtGeomFileName=TS-Encoder 2.0_Default_sldprt.STEP  UnitType=FromFile  ExtGeomFileUnits=m  StepReaderType=HEX  ExportConvexHullGeometry=off  InertiaType=CalculateFromGeometry  Mass=1  MassUnits=kg  CenterOfMass=[0 0 0]  CenterOfMassUnits=m  MomentsOfInertia=[1 1 1]  MomentsOfInertiaUnits=kg*m^2  ProductsOfInertia=[0 0 0]  ProductsOfInertiaUnits=kg*m^2  BasedOnType=Density  Density=1000  DensityUnits=kg/m^3  DoExposeReferenceFrame=off  SerializedFrames=<Frames><Frame><Id>Frame1</Id><Value><Name>F1</Name><Origin><Source>GeometricFeature</Source><FeatureName>planar surface 4</FeatureName></Origin><PrimaryAxis><DefinedDirection>+Z</DefinedDirection><Source>ReferenceFrame</Source><SourceDirection>+Z</SourceDirection><FeatureName></FeatureName></PrimaryAxis><SecondaryAxis><DefinedDirection>+X</DefinedDirection><Source>ReferenceFrame</Source><SourceDirection>+X</SourceDirection><FeatureName></FeatureName></SecondaryAxis></Value></Frame><Frame><Id>Frame2</Id><Value><Name>F2</Name><Origin><Source>GeometricFeature</Source><FeatureName>planar surface 11</FeatureName></Origin><PrimaryAxis><DefinedDirection>+Z</DefinedDirection><Source>ReferenceFrame</Source><SourceDirection>+Z</SourceDirection><FeatureName></FeatureName></PrimaryAxis><SecondaryAxis><DefinedDirection>+X</DefinedDirection><Source>ReferenceFrame</Source><SourceDirection>+X</SourceDirection><FeatureName></FeatureName></SecondaryAxis></Value></Frame></Frames>  GraphicType=FromGeometry  MarkerShape=Sphere  MarkerSize=10  GraphicVisPropType=SimpleVisualProperties  GraphicDiffuseColor=[0.4 0.4 0.4]  GraphicSpecularColor=[0.5 0.5 0.5 1.0]  GraphicAmbientColor=[0.15 0.15 0.15 1.0]  GraphicEmissiveColor=[0.0 0.0 0.0 1.0]  GraphicShininess=75  GraphicOpacity=1
  External Force and Torque : sm_lib/Forces and Torques/External Force and Torque  ForceResolutionFrame=AttachedFrame  EnableForceX=on  EnableForceY=off  EnableForceZ=off  EnableForce=off  TorqueResolutionFrame=AttachedFrame  EnableTorqueX=off  EnableTorqueY=off  EnableTorqueZ=off  EnableTorque=off
  Mechanism Configuration : sm_lib/Utilities/Mechanism Configuration  UniformGravity=Constant  GravityVector=[0 0 0]  GravityUnits=m/s^2  LinearizationDelta=0.001  JointModeTransitionNonlinearIterations=2
  PS-Simulink Converter : nesl_utility/PS-Simulink Converter  PhysicalDomain=network_engine_domain  SubClassName=ps_output  LeftPortType=input  RightPortType=output  PseudoPeriodic=off  Frequencies=[]  Unit=deg  AffineConversion=off
      settings: SourceProductBaseCode=PW,SS
  Revolute Joint : sm_lib/Joints/Revolute Joint  JointMode=Normal  SenseConstraintForce=off  SenseConstraintForceX=off  SenseConstraintForceY=off  SenseConstraintForceZ=off  SenseConstraintTorque=off  SenseConstraintTorqueX=off  SenseConstraintTorqueY=off  SenseConstraintTorqueZ=off  SenseTotalForce=off  SenseTotalForceX=off  SenseTotalForceY=off  SenseTotalForceZ=off  SenseTotalTorque=off  SenseTotalTorqueX=off  SenseTotalTorqueY=off  SenseTotalTorqueZ=off  CompositeWrenchDir=FollowerOnBase  CompositeWrenchFrame=BaseFrame  EquilibriumPosition=0  EquilibriumPositionUnits=deg  SpringStiffness=kt1  SpringStiffnessUnits=N*m/rad  DampingCoefficient=d  DampingCoefficientUnits=N*m/(deg/s)  TorqueActuationMode=NoTorque  MotionActuationMode=ComputedMotion  SensePosition=on  SenseVelocity=off  SenseAcceleration=off  SenseTorqueForce=off  SenseLowerLimitTorqueForce=off  SenseUpperLimitTorqueForce=off  LowerLimitSpecify=off  LowerLimitBound=-90  LowerLimitBoundUnits=deg  LowerLimitStiffness=1e4  LowerLimitStiffnessUnits=N*m/deg  LowerLimitDamping=10  LowerLimitDampingUnits=N*m/(deg/s)  LowerLimitTransitionRegionWidth=0.1  LowerLimitTransitionRegionWidthUnits=deg  UpperLimitSpecify=off  UpperLimitBound=90  UpperLimitBoundUnits=deg  UpperLimitStiffness=1e4  UpperLimitStiffnessUnits=N*m/deg  UpperLimitDamping=10  UpperLimitDampingUnits=N*m/(deg/s)  UpperLimitTransitionRegionWidth=0.1  UpperLimitTransitionRegionWidthUnits=deg  PositionTargetSpecify=on  PositionTargetPriority=High  PositionTargetValue=pos1  PositionTargetValueUnits=deg  VelocityTargetSpecify=off  VelocityTargetPriority=High  VelocityTargetValue=0  VelocityTargetValueUnits=deg/s
  Rigid Transform : sm_lib/Frames and Transforms/Rigid Transform  TranslationMethod=StandardAxis  TranslationStandardOffset=.3  TranslationLengthUnit=mm  TranslationStandardAxis=+Z  TranslationCartesianOffset=[0 0 0]  TranslationROffset=0  TranslationROffsetUnits=m  TranslationZOffset=0  TranslationZOffsetUnits=m  TranslationThetaOffset=0  TranslationThetaOffsetUnits=deg  RotationMethod=None  RotationAngleUnits=deg  RotationStandardAxis=+Z  RotationAngle=0.0  RotationArbitraryAxis=[0 0 1]  FollAlignAxisA=+X  BaseAlignAxisA=+Y  FollAlignAxisB=+Y  BaseAlignAxisB=+Z  RotationSequenceAxes=FollowerAxes  RotationSequence=XYX  RotationSequenceAngles=[0 0 0]  RotationSequenceAnglesUnits=deg  RotationMatrix=[1 0 0; 0 1 0; 0 0 1]
  Rigid Transform1 : sm_lib/Frames and Transforms/Rigid Transform  TranslationMethod=StandardAxis  TranslationStandardOffset=11  TranslationLengthUnit=mm  TranslationStandardAxis=+Z  TranslationCartesianOffset=[0 0 0]  TranslationROffset=0  TranslationROffsetUnits=m  TranslationZOffset=0  TranslationZOffsetUnits=m  TranslationThetaOffset=0  TranslationThetaOffsetUnits=deg  RotationMethod=None  RotationAngleUnits=deg  RotationStandardAxis=+Z  RotationAngle=0.0  RotationArbitraryAxis=[0 0 1]  FollAlignAxisA=+X  BaseAlignAxisA=+Y  FollAlignAxisB=+Y  BaseAlignAxisB=+Z  RotationSequenceAxes=FollowerAxes  RotationSequence=XYX  RotationSequenceAngles=[0 0 0]  RotationSequenceAnglesUnits=deg  RotationMatrix=[1 0 0; 0 1 0; 0 0 1]
  Rigid Transform2 : sm_lib/Frames and Transforms/Rigid Transform  Commented=on  TranslationMethod=StandardAxis  TranslationStandardOffset=dmass  TranslationLengthUnit=mm  TranslationStandardAxis=+X  TranslationCartesianOffset=[0 0 0]  TranslationROffset=0  TranslationROffsetUnits=m  TranslationZOffset=0  TranslationZOffsetUnits=m  TranslationThetaOffset=0  TranslationThetaOffsetUnits=deg  RotationMethod=None  RotationAngleUnits=deg  RotationStandardAxis=+Z  RotationAngle=0.0  RotationArbitraryAxis=[0 0 1]  FollAlignAxisA=+X  BaseAlignAxisA=+Y  FollAlignAxisB=+Y  BaseAlignAxisB=+Z  RotationSequenceAxes=FollowerAxes  RotationSequence=XYX  RotationSequenceAngles=[0 0 0]  RotationSequenceAnglesUnits=deg  RotationMatrix=[1 0 0; 0 1 0; 0 0 1]
  Rigid Transform3 : sm_lib/Frames and Transforms/Rigid Transform  TranslationMethod=StandardAxis  TranslationStandardOffset=ll-7  TranslationLengthUnit=mm  TranslationStandardAxis=+Z  TranslationCartesianOffset=[0 0 0]  TranslationROffset=0  TranslationROffsetUnits=m  TranslationZOffset=0  TranslationZOffsetUnits=m  TranslationThetaOffset=0  TranslationThetaOffsetUnits=deg  RotationMethod=None  RotationAngleUnits=deg  RotationStandardAxis=+Z  RotationAngle=0.0  RotationArbitraryAxis=[0 0 1]  FollAlignAxisA=+X  BaseAlignAxisA=+Y  FollAlignAxisB=+Y  BaseAlignAxisB=+Z  RotationSequenceAxes=FollowerAxes  RotationSequence=XYX  RotationSequenceAngles=[0 0 0]  RotationSequenceAnglesUnits=deg  RotationMatrix=[1 0 0; 0 1 0; 0 0 1]
  Scope : Scope
  Scope1 : Scope
  Simulink-PS Converter : nesl_utility/Simulink-PS Converter  PhysicalDomain=network_engine_domain  SubClassName=ps_input  LeftPortType=input  RightPortType=output  PseudoPeriodic=off  Frequencies=[]  NoiseDistribution=none  NoiseParameters=[]  Unit=N  AffineConversion=off  FilteringAndDerivatives=filter  SimscapeFilterOrder=2  InputFilterTimeConstant=0.001  UdotUserProvided=0
      settings: SourceProductBaseCode=PW,SS
  Sine Wave : Sin  Amplitude=Har_Force  Frequency=freq  SampleTime=0
  Solver Configuration : nesl_utility/Solver Configuration  PhysicalDomain=network_engine_domain  SubClassName=solver  LeftPortType=input  RightPortType=generic  Tones=[]  Harmonics=[]  SimulateNoise=off  Profile=off  UseLocalSampling=off  EnableSwitchedLinearOptims=on  FrequencyDomain=off  UseCCode=off  RelTol=0.001  AbsTol=1e-06  MinStep=1e-09  ToWorkspace=off  RevertToSquareIcSolve=off  NumHomotopyIterations=100  PhasorMode=off  PhasorModeNumHarmonics=1  DoDC=off  ResidualTolerance=1e-09  UseLocalSolver=off  LocalSolverChoice=NE_BACKWARD_EULER_ADVANCER  LocalSolverSampleTime=0.001  DoFixedCost=off  MaxNonlinIter=3  MaxModeIter=2  ComputeImpulses=off  ImpulseIterations=2  LinearAlgebra=Sparse  EquationFormulation=NE_TIME_EF  DelaysMemoryBudget=1024  AutomaticFiltering=on  FilteringTimeConstant=0.001  PartitionStorageMethod=AS_NEEDED  PartitionMemoryBudget=1024  PartitionMethod=FAST
      settings: SourceProductBaseCode=PW,SS
  Spring : sm_lib/Body Elements/File Solid  ExtGeomFileName=TS-Spring_Default_sldprt.STEP  UnitType=FromFile  ExtGeomFileUnits=m  StepReaderType=HEX  ExportConvexHullGeometry=off  InertiaType=CalculateFromGeometry  Mass=1  MassUnits=kg  CenterOfMass=[0 0 0]  CenterOfMassUnits=m  MomentsOfInertia=[1 1 1]  MomentsOfInertiaUnits=kg*m^2  ProductsOfInertia=[0 0 0]  ProductsOfInertiaUnits=kg*m^2  BasedOnType=Density  Density=b_den  DensityUnits=g/cm^3  DoExposeReferenceFrame=off  SerializedFrames=<Frames><Frame><Id>Frame1</Id><Value><Name>F1</Name><Origin><Source>GeometricFeature</Source><FeatureName>circular curve 1</FeatureName></Origin><PrimaryAxis><DefinedDirection>+Z</DefinedDirection><Source>ReferenceFrame</Source><SourceDirection>+Z</SourceDirection><FeatureName></FeatureName></PrimaryAxis><SecondaryAxis><DefinedDirection>+X</DefinedDirection><Source>ReferenceFrame</Source><SourceDirection>-Y</SourceDirection><FeatureName></FeatureName></SecondaryAxis></Value></Frame></Frames>  GraphicType=FromGeometry  MarkerShape=Sphere  MarkerSize=10  GraphicVisPropType=SimpleVisualProperties  GraphicDiffuseColor=[0.4 0.4 0.4]  GraphicSpecularColor=[0.5 0.5 0.5 1.0]  GraphicAmbientColor=[0.15 0.15 0.15 1.0]  GraphicEmissiveColor=[0.0 0.0 0.0 1.0]  GraphicShininess=75  GraphicOpacity=1
  Step : Step  Time=.1  Before=Force  After=0  SampleTime=0
  Subsystem : Subsystem
  Subsystem1 : Subsystem
      settings: PortSchema="{\"entries\":[{\"content\":{\"sides\":[{\"content\":{\"connectorIds\":[\"LConn1\"]},\"type\":\"ConnectorPlacement.EquallySpacedRectSide\",\"uuid\":\"d68d92a3-376a-4baf-a7a9-f6ce211c7a0e\"},{\"content\":{\"connectorIds\":[\"RConn1\"],\"side\":\"RIGHT\"},\"type\":\"ConnectorPlacement.EquallySpacedRectSide\",\"uuid\":\"ed7c6dd7-0ec9-44a8-a8c4-0583e8e4929e\"},{\"content\":{\"connectorIds\":[\"LConn2\"],\"side\":\"TOP\"},\"type\":\"ConnectorPlacement.EquallySpacedRectSide\",\"uuid\":\"19f7fd0e-0f62-423e-81aa-970ee34d1548\"}]},\"type\":\"ConnectorPlacement.EquallySpacedConnector\",\"uuid\":\"8f38fc93-c1f3-4589-b751-4b36a157facc\"}],\"packageUris\":[\"http://schema.mathworks.com/mf0/Connector/R2020b\"],\"version\":\"1.0\"}"
  Sum : Sum
  To Workspace : ToWorkspace  VariableName=disc1_pos  SampleTime=-1
  World Frame : sm_lib/Frames and Transforms/World Frame
  wires:
  PS-Simulink Converter/1 -> To Workspace/1, Scope1/1  "Disc 1"
  Sum/1 -> Simulink-PS Converter/1, Scope/1
  Step/1 -> Sum/1
  Sine Wave/1 -> Sum/2
  connections:
  Simulink-PS Converter/RConn1 -- External Force and Torque/LConn1
  PS-Simulink Converter/LConn1 -- Revolute Joint/RConn2
  World Frame/RConn1 -- Mechanism Configuration/RConn1 -- Subsystem/LConn1 -- Solver Configuration/RConn1
  Bracket2/LConn1 -- Subsystem/RConn2
  Spring/LConn1 -- Subsystem/RConn3
  Subsystem/RConn1 -- Bracket1/LConn1
  Bearing1/RConn1 -- Rigid Transform/LConn1
  Rigid Transform/RConn1 -- Revolute Joint/LConn1
  Encoder1/LConn1 -- Rigid Transform1/RConn1
  Rigid Transform3/RConn1 -- Bearing1/LConn1 -- Rigid Transform1/LConn1
  Rigid Transform3/LConn1 -- Bracket2/RConn1
  Subsystem1/RConn1 -- Revolute Joint/RConn1
  External Force and Torque/RConn1 -- Subsystem1/LConn1
  Cylindrical Solid/LConn1 -- Rigid Transform2/RConn1
  Rigid Transform2/LConn1 -- Subsystem1/LConn2
